simulink model "RRR_Dynamics"  (R2019b)
settings: Solver=ode3  StartTime=0.0  StopTime=30  FixedStep=0.01  RelTol=1e-3
undefined symbols (not defined in the file or in its folder): x_init
libraries: simulink x14
settings Model: Creator=Chris  LastModifiedBy=Chris

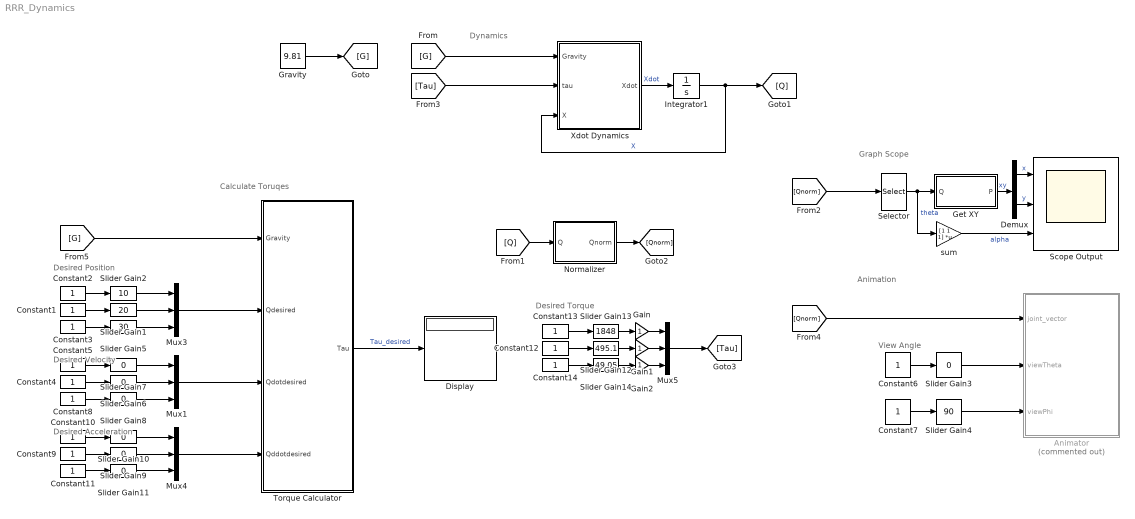
== system RRR_Dynamics ==
  note: Calculate Toruqes
  note: Dynamics
  note: Graph Scope
  note: Animation
  note: Desired Position
  note: View Angle
  note: Desired Velocity
  note: Desired Acceleration
  note: Desired Torque
  Animator : MATLAB Function  Commented=on  TreatAsAtomicUnit=on
  Constant{1..14} (14 alike) : Constant
  Demux : Demux  Outputs=2
  Display : Display
  Gain : Gain
  Gain1 : Gain
  Gain2 : Gain
  Get XY : MATLAB Function  TreatAsAtomicUnit=on
  Gravity : Constant  Value=9.81
  Integrator1 : Integrator  InitialCondition=-x_init
  Mux{1,3..5} (4 alike) : Mux  Inputs=3
  Normalizer : MATLAB Function  TreatAsAtomicUnit=on
  Scope Output : Scope  NumInputPorts=3
  Selector : Selector  InputPortWidth=6  IndexOptions=Index vector (dialog)  Indices=[1 3 5]  OutputSizes=1
  Slider Gain1 : simulink/Math Operations/Slider Gain  gain=20  low=-90  high=90
  Slider Gain{3,6..11} (7 alike) : simulink/Math Operations/Slider Gain  gain=0  low=-90  high=90
  Slider Gain12 : simulink/Math Operations/Slider Gain  gain=495.1  low=-5000  high=5000
  Slider Gain13 : simulink/Math Operations/Slider Gain  gain=1848  low=-5000  high=5000
  Slider Gain14 : simulink/Math Operations/Slider Gain  gain=49.05  low=-5000  high=5000
  Slider Gain2 : simulink/Math Operations/Slider Gain  gain=10  low=-90  high=90
  Slider Gain4 : simulink/Math Operations/Slider Gain  gain=90  low=-90  high=90
  Slider Gain5 : simulink/Math Operations/Slider Gain  gain=30  low=-90  high=90
  Torque Calculator : MATLAB Function  TreatAsAtomicUnit=on
  Xdot Dynamics : MATLAB Function  TreatAsAtomicUnit=on
  sum : Gain  Gain=[1 1 1]  Multiplication=Matrix(K*u)
  wires:
  Torque Calculator/1(Tau) -> Display/1  "Tau_desired"
  Mux3/1 -> Torque Calculator/2(Qdesired)
  Slider Gain5/1 -> Mux3/3
  Constant3/1 -> Slider Gain5/1
  Slider Gain1/1 -> Mux3/2
  Slider Gain2/1 -> Mux3/1
  Constant1/1 -> Slider Gain1/1
  Constant2/1 -> Slider Gain2/1
  Xdot Dynamics/1(Xdot) -> Integrator1/1  "Xdot"
  Slider Gain3/1 -> Animator/2(viewTheta)
  Slider Gain4/1 -> Animator/3(viewPhi)
  Constant6/1 -> Slider Gain3/1
  Constant7/1 -> Slider Gain4/1
  Slider Gain7/1 -> Mux1/1
  Constant8/1 -> Slider Gain8/1
  Slider Gain8/1 -> Mux1/3
  Slider Gain6/1 -> Mux1/2
  Constant4/1 -> Slider Gain6/1
  Constant5/1 -> Slider Gain7/1
  Mux1/1 -> Torque Calculator/3(Qdotdesired)
  Constant9/1 -> Slider Gain9/1
  Slider Gain10/1 -> Mux4/1
  Slider Gain11/1 -> Mux4/3
  Constant10/1 -> Slider Gain10/1
  Slider Gain9/1 -> Mux4/2
  Mux4/1 -> Torque Calculator/4(Qddotdesired)
  Constant11/1 -> Slider Gain11/1
  Gravity/1 -> [G]
  [G] -> Xdot Dynamics/1(Gravity)
  Integrator1/1 -> Xdot Dynamics/3(X), [Q]  "X"
  [Qnorm] -> Selector/1
  Mux5/1 -> [Tau]
  Constant13/1 -> Slider Gain13/1
  Slider Gain13/1 -> Gain/1
  Constant12/1 -> Slider Gain12/1
  Slider Gain12/1 -> Gain1/1
  Constant14/1 -> Slider Gain14/1
  Slider Gain14/1 -> Gain2/1
  [Tau] -> Xdot Dynamics/2(tau)
  [Qnorm] -> Animator/1(joint_vector)
  [G] -> Torque Calculator/1(Gravity)
  Normalizer/1(Qnorm) -> [Qnorm]
  [Q] -> Normalizer/1(Q)
  sum/1 -> Scope Output/3  "alpha"
  Selector/1 -> sum/1, Get XY/1(Q)  "theta"
  Gain/1 -> Mux5/1
  Gain1/1 -> Mux5/2
  Gain2/1 -> Mux5/3
  Get XY/1(P) -> Demux/1  "xy"
  Demux/1 -> Scope Output/1  "x"
  Demux/2 -> Scope Output/2  "y"

== matlab function RRR_Dynamics/Normalizer ==
  data: Q input; Qnorm output
function Qnorm = fcn(Q)

q = Q(1:3);
qdot = Q(4:6);
qnorm = 2.*atan(tan(q./2));

Qnorm = [qnorm;qdot];

== matlab function RRR_Dynamics/Xdot Dynamics ==
  data: Xdot output; Gravity input; tau input; X input
function Xdot = xdot(Gravity,tau,X)

%% Unpack Variables
SFric1=0;
DFric1=200;
SFric2=0;
DFric2=150;
SFric3=0;
DFric3=100;

grav=Gravity;

q1=X(1);
q1dot=X(2);
q2=X(3);
q2dot=X(4);
q3=X(5);
q3dot=X(6);

%% Calculate Dynamics Matrices
Mq = [...
      80*cos(q2 + q3) + 420*cos(q2) + 60*cos(q3) + 12291/20, 40*cos(q2 + q3) + 210*cos(q2) + 60*cos(q3) + 2681/20, 40*cos(q2 + q3) + 30*cos(q3) + 101/10;...
       40*cos(q2 + q3) + 210*cos(q2) + 60*cos(q3) + 2681/20,                                 60*cos(q3) + 2681/20,                   30*cos(q3) + 101/10;...
                      40*cos(q2 + q3) + 30*cos(q3) + 101/10,                                  30*cos(q3) + 101/10,                                101/10;...
];


Vq = [...
      - q3dot*(40*q2dot*sin(q2 + q3) + q3dot*(40*sin(q2 + q3) + 30*sin(q3))) - q2dot*(q3dot*(40*sin(q2 + q3) + 60*sin(q3)) + q2dot*(40*sin(q2 + q3) + 210*sin(q2))) - q1dot*(q3dot*(80*sin(q2 + q3) + 60*sin(q3)) + q2dot*(80*sin(q2 + q3) + 420*sin(q2)));...
      210*q1dot^2*sin(q2) - 30*q3dot^2*sin(q3) + 40*q1dot^2*sin(q2 + q3) - 60*q1dot*q3dot*sin(q3) - 60*q2dot*q3dot*sin(q3);...
      30*q1dot^2*sin(q3) + 30*q2dot^2*sin(q3) + 40*q1dot^2*sin(q2 + q3) + 60*q1dot*q2dot*sin(q3);...
];

Gq = [...
      (5*grav*(4*cos(q1 + q2 + q3) + 21*cos(q1 + q2) + 56*cos(q1)))/2;...
      (105*grav*cos(q1 + q2))/2 + 10*grav*cos(q1 + q2 + q3);...
      10*grav*cos(q1 + q2 + q3);...
];


F1=SFric1*sign(q1dot) + DFric1*q1dot;
F2=SFric2*sign(q2dot) + DFric2*q2dot;
F3=SFric3*sign(q3dot) + DFric3*q3dot;

Fq=[F1;F2;F3];

%% Get Acceleration and Xdot
accel = Mq^(-1)*(tau - Vq - Gq - Fq);
Xdot=[q1dot;accel(1);q2dot;accel(2);q3dot;accel(3)];


end

== matlab function RRR_Dynamics/Animator ==
  data: joint_vector input; viewTheta input; viewPhi input
function Model_Robot(joint_vector, viewTheta, viewPhi)

%% Unpack Joint Vector
theta = joint_vector;
L1 = 8;
L2 = 6;
EOA = 4;
L = [0 L1 L2 EOA];

%% Define Links/ Robot Shapes
origin = [0;0;0];

Base  = [...
         -1  -1  -1  -1  -1   1   1  -1   1   1  -1   1   1  -1   1   1;...
          1  -1  -1   1   1   1   1   1   1  -1  -1  -1  -1  -1  -1   1;...
        -15 -15  -1  -1 -15 -15  -1  -1  -1  -1  -1  -1 -15 -15 -15 -15;...
];

Link1 = [...
          1  -1  -1   1   1   1   1   1   1  -1  -1  -1  -1  -1  -1   1;...
          1   1  -1  -1   1   1  -1  -1  -1  -1  -1  -1   1   1   1   1;...
         -1  -1  -1  -1  -1   1   1  -1   1   1  -1   1   1  -1   1   1;...
];

L1rod = [...
          1  L1  L1   1   1   1   1   1   1  L1  L1  L1  L1  L1  L1   1;...
         .5  .5 -.5 -.5  .5  .5 -.5 -.5 -.5 -.5 -.5 -.5  .5  .5  .5  .5;...
        -.5 -.5 -.5 -.5 -.5  .5  .5 -.5  .5  .5 -.5  .5  .5 -.5  .5  .5;...
];

Link2 = [...
          1  -1  -1   1   1   1   1   1   1  -1  -1  -1  -1  -1  -1   1;...
          1   1  -1  -1   1   1  -1  -1  -1  -1  -1  -1   1   1   1   1;...
         -1  -1  -1  -1  -1   1   1  -1   1   1  -1   1   1  -1   1   1;...
];

L2rod = [...
          1  L2  L2   1   1   1   1   1   1  L2  L2  L2  L2  L2  L2   1;...
         .5  .5 -.5 -.5  .5  .5 -.5 -.5 -.5 -.5 -.5 -.5  .5  .5  .5  .5;...
        -.5 -.5 -.5 -.5 -.5  .5  .5 -.5  .5  .5 -.5  .5  .5 -.5  .5  .5;...
];

Link3 = [...
          1  -1  -1   1   1   1   1   1   1  -1  -1  -1  -1  -1  -1   1;...
          1   1  -1  -1   1   1  -1  -1  -1  -1  -1  -1   1   1   1   1;...
         -1  -1  -1  -1  -1   1   1  -1   1   1  -1   1   1  -1   1   1;...
];

L3rod = [...
          1  EOA EOA  1   1   1   1   1   1  EOA EOA EOA EOA EOA EOA  1;...
         .5  .5 -.5 -.5  .5  .5 -.5 -.5 -.5 -.5 -.5 -.5  .5  .5  .5  .5;...
        -.5 -.5 -.5 -.5 -.5  .5  .5 -.5  .5  .5 -.5  .5  .5 -.5  .5  .5;...
];

% shape of axis figure for base and EOAT
axes  = [...
         0 1.5 0  0  0  0  0;...
         0  0  0 1.5 0  0  0;...
         0  0  0  0  0 1.5 0;...
];

%% Transform Link 1
BaseLink1= TRANSRRR(Link1 ,theta(1), L(1));
Link1rod = TRANSRRR(L1rod ,theta(1), L(1));

%% Transform Link 2
Link12   = TRANSRRR(Link2 ,theta(2), L(2));
BaseLink2= TRANSRRR(Link12,theta(1), L(1));

L2rod    = TRANSRRR(L2rod ,theta(2), L(2));
Link2rod = TRANSRRR(L2rod ,theta(1), L(1));
% BaseLink2O = TRANS01SF(TRANS12SF(origin,theta2),theta1);

%% Transform Link 3
Link23   = TRANSRRR(Link3 ,theta(3), L(3));
Link13   = TRANSRRR(Link23,theta(2), L(2));
BaseLink3= TRANSRRR(Link13,theta(1), L(1));

L3rod    = TRANSRRR(L3rod ,theta(3), L(3));
L3rod    = TRANSRRR(L3rod ,theta(2), L(2));
Link3rod = TRANSRRR(L3rod ,theta(1), L(1));
% BaseLink3O = TRANS01SF(TRANS12SF(TRANS23SF(origin,d3),theta2),theta1);


%% Plotting
plot3(Base(1,:),Base(2,:),Base(3,:),'k-')
axis([-20 20 -20 20 -20 20]);
grid on
hold on
plot3(BaseLink1(1,:),BaseLink1(2,:),BaseLink1(3,:),'b-', 'LineWidth', 2)
plot3(Link1rod(1,:), Link1rod(2,:), Link1rod(3,:), 'b-', 'LineWidth', 2)
plot3(BaseLink2(1,:),BaseLink2(2,:),BaseLink2(3,:),'g-', 'LineWidth', 2)
plot3(Link2rod(1,:), Link2rod(2,:), Link2rod(3,:), 'g-', 'LineWidth', 2)
plot3(BaseLink3(1,:),BaseLink3(2,:),BaseLink3(3,:),'k-', 'LineWidth', 2)
plot3(Link3rod(1,:), Link3rod(2,:), Link3rod(3,:), 'k-', 'LineWidth', 2)

xlabel('X');
ylabel('Y');
zlabel('Z');
view(viewTheta,viewPhi);
set(gcf,'color','w');
hold off

end

== matlab function RRR_Dynamics/Torque Calculator ==
  data: Tau output; Gravity input; Qdesired input; Qdotdesired input; Qddotdesired input
function Tau = tau_calc(Gravity,Qdesired,Qdotdesired,Qddotdesired)

SFric1=0;
DFric1=200;
SFric2=0;
DFric2=150;
SFric3=0;
DFric3=100;

grav=Gravity;

q1 = Qdesired(1)*pi/180;
q2 = Qdesired(2)*pi/180;
q3 = Qdesired(3)*pi/180;
q1dot = Qdotdesired(1);
q2dot = Qdotdesired(2);
q3dot = Qdotdesired(3);
q1ddot = Qddotdesired(1);
q2ddot = Qddotdesired(2);
q3ddot = Qddotdesired(3);



Mq = [...
      80*cos(q2 + q3) + 420*cos(q2) + 60*cos(q3) + 12291/20, 40*cos(q2 + q3) + 210*cos(q2) + 60*cos(q3) + 2681/20, 40*cos(q2 + q3) + 30*cos(q3) + 101/10;...
       40*cos(q2 + q3) + 210*cos(q2) + 60*cos(q3) + 2681/20,                                 60*cos(q3) + 2681/20,                   30*cos(q3) + 101/10;...
                      40*cos(q2 + q3) + 30*cos(q3) + 101/10,                                  30*cos(q3) + 101/10,                                101/10;...
];


Vq = [...
      - q3dot*(40*q2dot*sin(q2 + q3) + q3dot*(40*sin(q2 + q3) + 30*sin(q3))) - q2dot*(q3dot*(40*sin(q2 + q3) + 60*sin(q3)) + q2dot*(40*sin(q2 + q3) + 210*sin(q2))) - q1dot*(q3dot*(80*sin(q2 + q3) + 60*sin(q3)) + q2dot*(80*sin(q2 + q3) + 420*sin(q2)));...
      210*q1dot^2*sin(q2) - 30*q3dot^2*sin(q3) + 40*q1dot^2*sin(q2 + q3) - 60*q1dot*q3dot*sin(q3) - 60*q2dot*q3dot*sin(q3);...
      30*q1dot^2*sin(q3) + 30*q2dot^2*sin(q3) + 40*q1dot^2*sin(q2 + q3) + 60*q1dot*q2dot*sin(q3);...
];

Gq = [...
      (5*grav*(4*cos(q1 + q2 + q3) + 21*cos(q1 + q2) + 56*cos(q1)))/2;...
      (105*grav*cos(q1 + q2))/2 + 10*grav*cos(q1 + q2 + q3);...
      10*grav*cos(q1 + q2 + q3);...
];


F1=SFric1*sign(q1dot) + DFric1*q1dot;
F2=SFric2*sign(q2dot) + DFric2*q2dot;
F3=SFric3*sign(q3dot) + DFric3*q3dot;


Fq=[F1;F2;F3];

Tau = Vq + Gq + Fq + Mq*[q1ddot;q2ddot;q3ddot];

end

== matlab function RRR_Dynamics/Get XY ==
  data: Q input; P output
function P   = TRANSRRR04(Q)

q1 = Q(1);
q2 = Q(2);
q3 = Q(3);

T01 = [...
       cos(q1)  -sin(q1)  0  0 ;...
       sin(q1)   cos(q1)  0  0 ;...
         0         0      1  0 ;...
         0         0      0  1 ;...
];


T12 = [...
       cos(q2)  -sin(q2)  0  4 ;...
       sin(q2)   cos(q2)  0  0 ;...
         0         0      1  0 ;...
         0         0      0  1 ;...
];

T23 = [...
       cos(q3)  -sin(q3)  0  3 ;...
       sin(q3)   cos(q3)  0  0 ;...
         0         0      1  0 ;...
         0         0      0  1 ;...
];

T34 = [...
         1         0      0  2 ;...
         0         1      0  0 ;...
         0         0      1  0 ;...
         0         0      0  1 ;...
];

T04 = T01*T12*T23*T34;
Pt = T04*[0;0;0;1];
P = [Pt(1); Pt(2)];
end
